simulink model "sf_bridge"  (R2017b)
settings: Solver=ode45  StartTime=0.0  StopTime=inf  RelTol=1e-3  EnableMultiTasking=on
libraries: sf_bidder x4
CloseFcn:
  | delete(findall(0, 'type', 'figure', 'tag', 'SF_BRIDGE'));
settings Model: FPTRunName=Active  ExtModeAutoUpdateStatusClock=off  Creator=The MathWorks, Inc.  LastModifiedBy=The MathWorks, Inc.
settings DataIOCC: LimitDataPoints=on  SaveFormat=Array  SignalLoggingName=sigsOut
settings OptimizationCC: ExpressionDepthLimit=2147483647  InitFltsAndDblsToZero=on  LifeSpan=inf
settings DebuggingCC: SaveWithParameterizedLinksMsg=none  UnderspecifiedInitializationDetection=Classic  MergeDetectMultiDrivingBlocksExec=none  CheckExecutionContextPreStartOutputMsg=on  CheckExecutionContextRuntimeOutputMsg=on  SignalResolutionControl=TryResolveAllWithWarning  MultiTaskDSMMsg=warning  MultiTaskCondExecSysMsg=none  FcnCallInpInsideContextMsg=warning  StateNameClashWarn=warning  StrictBusMsg=None  SFUnexpectedBacktrackingDiag=warning  SFNoUnconditionalDefaultTransitionDiag=warning  SFExecutionAtInitializationDiag=none
settings HardwareCC: ProdBitPerPointer=32  ProdBitPerSizeT=32  ProdBitPerPtrDiffT=32  ProdLargestAtomicFloat=None  ProdIntDivRoundTo=Undefined  ProdEndianess=Unspecified  ProdWordSize=32  ProdHWDeviceType=32-bit Generic  TargetUnknown=on
settings ModelReferenceCC: PropagateSignalLabelsOutOfModel=off
settings SFSimCC: SimParseCustomCode=off
settings CodeAppCC: StateflowObjectComments=on
settings GRTTargetCC: TargetFcnLib=ansi_tfl_tmw.mat  TargetLangStandard=C89/C90 (ANSI)  GeneratePreprocessorConditionals=Disable all  CombineOutputUpdateFcns=off  GRTInterface=on
settings ConfigComp: CovMetricSettings=dcmtr  CovHtmlReporting=on  CovSaveCumulativeToWorkspaceVar=on  CovSaveSingleToWorkspaceVar=on  CovExternalEMLEnable=off  CovSFcnEnable=off

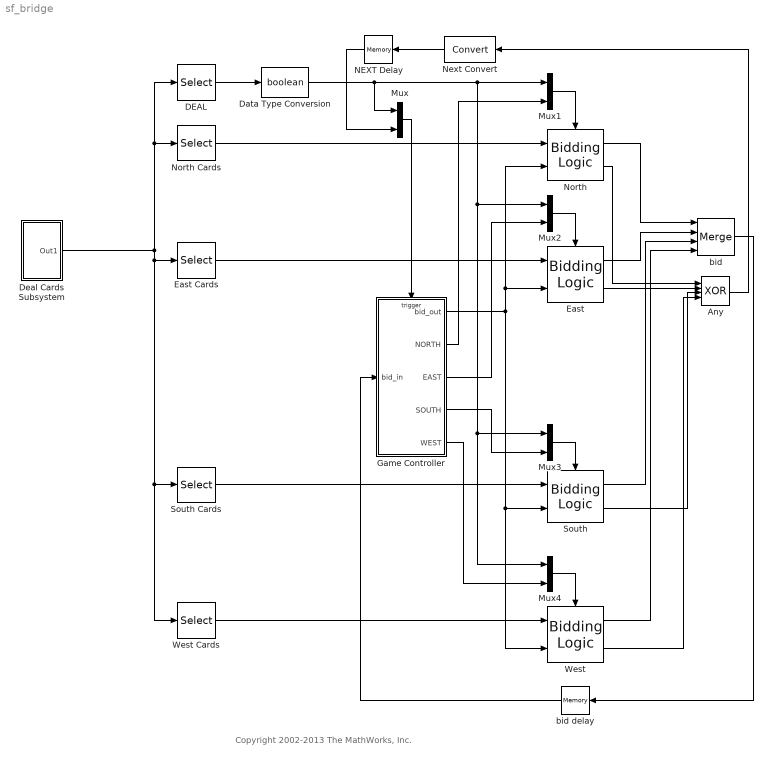
== system sf_bridge ==
  note: Copyright 2002-2013 The MathWorks, Inc.
  Any : Logic  Operator=XOR  Inputs=4  AllPortsSameDT=off
  DEAL : Selector  InputPortWidth=53  IndexOptions=Index vector (dialog)  Indices=[1]  OutputSizes=1
  Data Type Conversion : DataTypeConversion  OutDataTypeStr=boolean
  Deal Cards Subsystem : Subsystem
  East : sf_bidder/Bidding Logic
      settings: SourceProductName=Stateflow  SourceProductBaseCode=SF
  East Cards : Selector  InputPortWidth=53  IndexOptions=Index vector (dialog)  Indices=[15:27]  OutputSizes=1
  Game Controller : Stateflow chart  TreatAsAtomicUnit=on
  Mux{,1..4} (5 alike) : Mux  Inputs=2
  NEXT Delay : Memory
  Next Convert : DataTypeConversion  SaturateOnIntegerOverflow=on  RndMeth=Zero
  North : sf_bidder/Bidding Logic
      settings: SourceProductName=Stateflow  SourceProductBaseCode=SF
  North Cards : Selector  InputPortWidth=53  IndexOptions=Index vector (dialog)  Indices=[2:14]  OutputSizes=1
  South : sf_bidder/Bidding Logic
      settings: SourceProductName=Stateflow  SourceProductBaseCode=SF
  South Cards : Selector  InputPortWidth=53  IndexOptions=Index vector (dialog)  Indices=[28:40]  OutputSizes=1
  West : sf_bidder/Bidding Logic
      settings: SourceProductName=Stateflow  SourceProductBaseCode=SF
  West Cards : Selector  InputPortWidth=53  IndexOptions=Index vector (dialog)  Indices=[41:53]  OutputSizes=1
  bid : Merge  Inputs=4
  bid delay : Memory
  wires:
  Deal Cards Subsystem/1(Out1) -> DEAL/1, North Cards/1, West Cards/1, South Cards/1, East Cards/1
  DEAL/1 -> Data Type Conversion/1
  bid/1 -> bid delay/1
  Any/1 -> Next Convert/1
  North Cards/1 -> North/1
  East Cards/1 -> East/1
  South Cards/1 -> South/1
  West Cards/1 -> West/1
  Game Controller/1(bid_out) -> South/2, West/2, North/2, East/2
  North/1 -> bid/1
  East/1 -> bid/2
  South/1 -> bid/3
  West/1 -> bid/4
  bid delay/1 -> Game Controller/1(bid_in)
  NEXT Delay/1 -> Mux/2
  Mux/1 -> Game Controller/Trigger
  North/2 -> Any/1
  West/2 -> Any/4
  East/2 -> Any/2
  South/2 -> Any/3
  Next Convert/1 -> NEXT Delay/1
  Mux1/1 -> North/Trigger
  Mux2/1 -> East/Trigger
  Mux3/1 -> South/Trigger
  Mux4/1 -> West/Trigger
  Game Controller/2(NORTH) -> Mux1/2
  Game Controller/3(EAST) -> Mux2/2
  Game Controller/4(SOUTH) -> Mux3/2
  Game Controller/5(WEST) -> Mux4/2
  Data Type Conversion/1 -> Mux/1, Mux1/1, Mux2/1, Mux4/1, Mux3/1

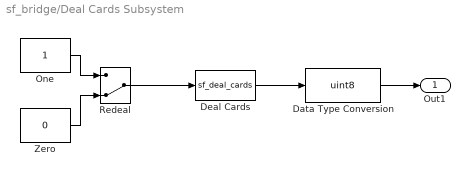
== system sf_bridge/Deal Cards Subsystem ==
  Data Type Conversion : DataTypeConversion  OutDataTypeStr=uint8
  Deal Cards : MATLABFcn  MATLABFcn=sf_deal_cards  OutputDimensions=53
  One : Constant
  Redeal : ManualSwitch  CurrentSetting=0
  Zero : Constant  Value=0
  Out1 : Outport
  wires:
  Redeal/1 -> Deal Cards/1
  One/1 -> Redeal/1
  Zero/1 -> Redeal/2
  Deal Cards/1 -> Data Type Conversion/1
  Data Type Conversion/1 -> Out1/1

== stateflow chart sf_bridge/Game Controller ==
  state Bidder [parallel]
    settings: executionOrder=1
    state North
      NORTH;
    state East
      EAST;
    state Done
    state South
      SOUTH;
    state West
      WEST;
    Done -> Bidder.North [order 2] : N_DEAL
    Bidder.West -> Bidder.North : NEXT_BID
    Bidder.North -> Bidder.East : NEXT_BID
    Bidder -> (junction 44) [order 1] : BID
        | {process_bid();}
    Done -> Bidder.East [order 1] : E_DEAL
    (default) -> Done
    Bidder.East -> Bidder.South : NEXT_BID
    Bidder -> Done [order 2] : ALL_PASS
        | {ml.sf_bridge_state('all_pass');}
    Done -> Bidder.South [order 4] : S_DEAL
    Done -> Bidder.West [order 3] : W_DEAL
    Bidder.South -> Bidder.West : NEXT_BID
    Bidder -> (junction 38) [order 3] : DEAL
        | {pass_count = 0;
        | bid_out = 0;}
  state process_bid() [function]
    (default) -> (junction 39) : {ml.sf_bridge_state('bid', bid_in);}
    (junction 39) -> (junction 41) [order 1] : [bid_in]
        | {pass_count = 0;
        | bid_out = bid_in;
        | send(NEXT_BID, Bidder);}
    (junction 39) -> (junction 42) [order 2] : {pass_count++;}
    (junction 42) -> (junction 46) [order 3] : {send(NEXT_BID, Bidder);}
    (junction 42) -> (junction 45) [order 1] : [pass_count == 4]
        | {send(ALL_PASS, Bidder);}
    (junction 42) -> (junction 43) [order 2] : [pass_count == 3]
    (junction 43) -> (junction 40) [order 1] : [bid_out]
        | {send(ALL_PASS,Bidder);}
    (junction 43) -> (junction 47) [order 2] : {send(NEXT_BID, Bidder);}
  state Dealer [parallel]
    settings: executionOrder=2
    state North
      ml.sf_bridge_state('deal', 'North');
      send(N_DEAL, Bidder);
    state East
      ml.sf_bridge_state('deal', 'East');
      send(E_DEAL, Bidder);
    state West
      ml.sf_bridge_state('deal', 'West');
      send(W_DEAL, Bidder);
    state South
      ml.sf_bridge_state('deal', 'South');
      send(S_DEAL, Bidder);
    (default) -> Dealer.North
    Dealer.West -> Dealer.North : DEAL
    Dealer.North -> Dealer.East : DEAL
    Dealer.East -> Dealer.South : DEAL
    Dealer.South -> Dealer.West : DEAL
  data: bid_in input uint8 size=1; bid_out output uint8 size=1; pass_count local uint8 size=1
  events: DEAL input EITHER_EDGE_EVENT; NORTH output EITHER_EDGE_EVENT; EAST output EITHER_EDGE_EVENT; SOUTH output EITHER_EDGE_EVENT; WEST output EITHER_EDGE_EVENT; BID input EITHER_EDGE_EVENT; E_DEAL local EITHER_EDGE_EVENT; NEXT_BID local EITHER_EDGE_EVENT; N_DEAL local EITHER_EDGE_EVENT; S_DEAL local EITHER_EDGE_EVENT; W_DEAL local EITHER_EDGE_EVENT; ALL_PASS local EITHER_EDGE_EVENT
